simulink model "flyingcap3lvl"  (R2023b)
settings: Solver=ode4  StartTime=0.0  StopTime=0.1  FixedStep=1e-5  RelTol=1e-3  EnableMultiTasking=on
libraries: spsIGBTDiodeLib x12, spsSeriesRLCBranchLib x8, simulink x6, spsVoltageMeasurementLib x4, spsCurrentMeasurementLib x3, spsGroundLib x2, spsDCVoltageSourceLib x1, spsThreePhaseVIMeasurementLib x1, spspowerguiLib x1
settings Model: Creator=Ranit  LastModifiedBy=user
settings SolverCC: AlgebraicLoopSolver=TrustRegion
settings DataIOCC: ReturnWorkspaceOutputs=off
settings OptimizationCC: LifeSpan=inf
settings DebuggingCC: UnconnectedInputMsg=warning  UnconnectedOutputMsg=warning  UnconnectedLineMsg=warning  SFUnexpectedBacktrackingDiag=warning  SFNoUnconditionalDefaultTransitionDiag=warning  ArithmeticOperatorsInVariantConditions=warning
settings ModelReferenceCC: EnableRefExpFcnMdlSchedulingChecks=on
settings SFSimCC: SimUseLocalCustomCode=off  CustomCodeUndefinedFunction=UseInterfaceOnly
settings RTWCC: RTWUseLocalCustomCode=off
settings CodeAppCC: StateflowObjectComments=on
settings GRTTargetCC: TargetLangStandard=C89/C90 (ANSI)
settings ConfigComp: CovMetricSettings=dw  CovSaveCumulativeToWorkspaceVar=on  CovSaveSingleToWorkspaceVar=on  CovExternalEMLEnable=off
settings SimscapeCC: SimscapeNormalizeSystem=off

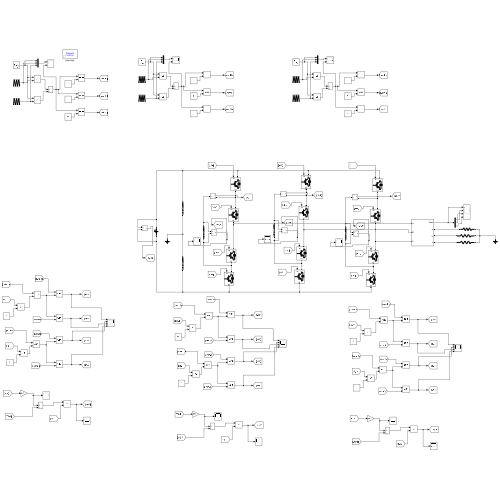
[thumbnail: Simulink's stored preview of the top-level diagram]
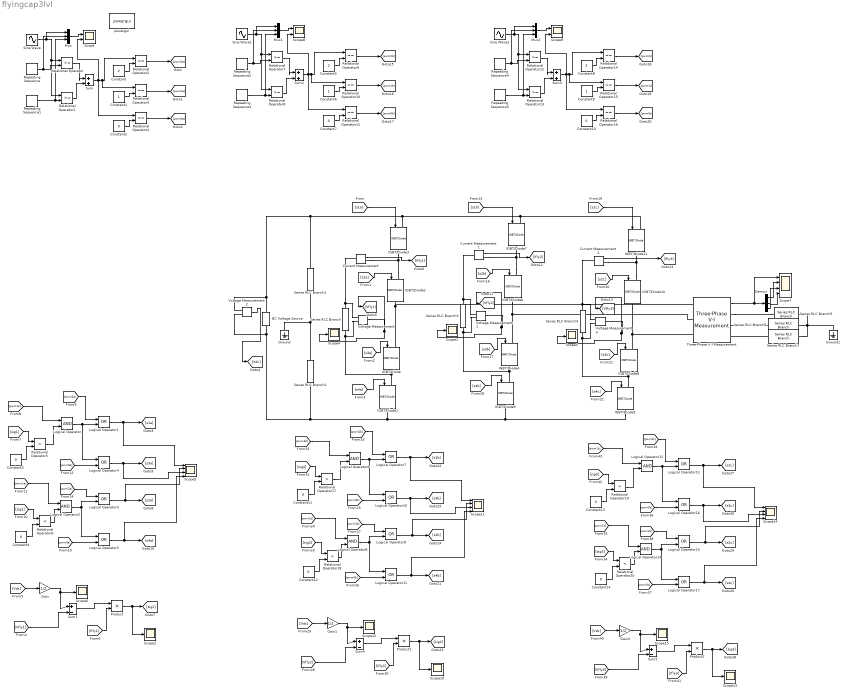
== system flyingcap3lvl ==
  Constant : Constant  Value=2
  Constant1 : Constant
  Constant{2..4,7,10..14} (9 alike) : Constant  Value=0
  Constant5 : Constant  Value=2
  Constant6 : Constant
  Constant8 : Constant  Value=2
  Constant9 : Constant
  Current Measurement : spsCurrentMeasurementLib/Current Measurement  PhasorSimulation=off  OutputType=Complex  PSBequivalent=0
  Current Measurement1 : spsCurrentMeasurementLib/Current Measurement  PhasorSimulation=off  OutputType=Complex  PSBequivalent=0
  Current Measurement2 : spsCurrentMeasurementLib/Current Measurement  PhasorSimulation=off  OutputType=Complex  PSBequivalent=0
  DC Voltage Source : spsDCVoltageSourceLib/DC Voltage Source  Amplitude=100  Measurements=None
  Demux : Demux  Outputs=3
  Gain : Gain  Gain=1/2
  Gain1 : Gain  Gain=1/2
  Gain2 : Gain  Gain=1/2
  Ground : spsGroundLib/Ground  LConnTagsString=a
  Ground1 : spsGroundLib/Ground  LConnTagsString=a
  IGBT/Diode{,1..11} (12 alike) : spsIGBTDiodeLib/IGBT//Diode  Ron=1e-3  Rs=1e5  Cs=inf  Measurements=off
  Logical Operator{,2,6,8,12,14} (6 alike) : Logic  AllPortsSameDT=off  OutDataTypeStr=boolean
  Logical Operator{1,3..5,7,9..11,13,15..17} (12 alike) : Logic  Operator=OR  AllPortsSameDT=off  OutDataTypeStr=boolean
  Mux : Mux  Inputs=3
  Mux1 : Mux  Inputs=3
  Mux2 : Mux  Inputs=3
  Product : Product
  Product1 : Product
  Product2 : Product
  Relational Operator{,1,7..8,12..13} (6 alike) : RelationalOperator  OutDataTypeStr=boolean  InputSameDT=off
  Relational Operator{2..4,9..11,14..16} (9 alike) : RelationalOperator  Operator===  OutDataTypeStr=boolean  InputSameDT=off
  Relational Operator17 : RelationalOperator  Operator=>  OutDataTypeStr=boolean  InputSameDT=off
  Relational Operator18 : RelationalOperator  Operator=<  OutDataTypeStr=boolean  InputSameDT=off
  Relational Operator19 : RelationalOperator  Operator=>  OutDataTypeStr=boolean  InputSameDT=off
  Relational Operator20 : RelationalOperator  Operator=<  OutDataTypeStr=boolean  InputSameDT=off
  Relational Operator5 : RelationalOperator  Operator=>  OutDataTypeStr=boolean  InputSameDT=off
  Relational Operator6 : RelationalOperator  Operator=<  OutDataTypeStr=boolean  InputSameDT=off
  Repeating Sequence : simulink/Sources/Repeating Sequence  rep_seq_t=[0 1 2]*[1/10000]  rep_seq_y=[0 1 0]
  Repeating Sequence1 : simulink/Sources/Repeating Sequence  rep_seq_t=[0 1 2]*[1/10000]  rep_seq_y=[-1 0 -1]
  Repeating Sequence2 : simulink/Sources/Repeating Sequence  rep_seq_t=[0 1 2]*[1/10000]  rep_seq_y=[0 1 0]
  Repeating Sequence3 : simulink/Sources/Repeating Sequence  rep_seq_t=[0 1 2]*[1/10000]  rep_seq_y=[-1 0 -1]
  Repeating Sequence4 : simulink/Sources/Repeating Sequence  rep_seq_t=[0 1 2]*[1/10000]  rep_seq_y=[0 1 0]
  Repeating Sequence5 : simulink/Sources/Repeating Sequence  rep_seq_t=[0 1 2]*[1/10000]  rep_seq_y=[-1 0 -1]
  Scope : Scope  NumInputPorts=2
  Scope{1..4,6,10,12..13,15} (9 alike) : Scope
  Scope{5,7,11,14} (4 alike) : Scope  NumInputPorts=4
  Scope8 : Scope  NumInputPorts=2
  Scope9 : Scope  NumInputPorts=2
  Series RLC Branch{,2..4} (4 alike) : spsSeriesRLCBranchLib/Series RLC Branch  LConnTagsString=__new0  RConnTagsString=__new0  BranchType=RC  Resistance=0.1  Inductance=1e-3  SetiL0=off  InitialCurrent=0  Capacitance=4.7e-3  Setx0=off  InitialVoltage=0  Measurements=None
  Series RLC Branch1 : spsSeriesRLCBranchLib/Series RLC Branch  LConnTagsString=__new0  RConnTagsString=__new0  BranchType=RC  Resistance=0.01  Inductance=1e-3  SetiL0=off  InitialCurrent=0  Capacitance=4.7e-3  Setx0=off  InitialVoltage=0  Measurements=None
  Series RLC Branch5 : spsSeriesRLCBranchLib/Series RLC Branch  LConnTagsString=__new0  RConnTagsString=__new0  BranchType=R  Resistance=500  Inductance=1e-3  SetiL0=off  InitialCurrent=0  Capacitance=1e-6  Setx0=off  InitialVoltage=0  Measurements=Branch voltage
  Series RLC Branch6 : spsSeriesRLCBranchLib/Series RLC Branch  LConnTagsString=__new0  RConnTagsString=__new0  BranchType=R  Resistance=100  Inductance=1e-3  SetiL0=off  InitialCurrent=0  Capacitance=1e-6  Setx0=off  InitialVoltage=0  Measurements=Branch voltage
  Series RLC Branch7 : spsSeriesRLCBranchLib/Series RLC Branch  LConnTagsString=__new0  RConnTagsString=__new0  BranchType=R  Resistance=250  Inductance=1e-3  SetiL0=off  InitialCurrent=0  Capacitance=1e-6  Setx0=off  InitialVoltage=0  Measurements=Branch voltage
  Sine Wave : Sin  Frequency=2*pi*50  SampleTime=0
  Sine Wave1 : Sin  Frequency=2*pi*50  Phase=4*pi/3  SampleTime=0
  Sine Wave2 : Sin  Frequency=2*pi*50  Phase=2*pi/3  SampleTime=0
  Sum : Sum  Inputs=|++
  Sum1 : Sum  Inputs=|+-
  Sum2 : Sum  Inputs=|++
  Sum3 : Sum  Inputs=|++
  Sum4 : Sum  Inputs=|+-
  Sum5 : Sum  Inputs=|+-
  Three-Phase V-I Measurement : spsThreePhaseVIMeasurementLib/Three-Phase V-I Measurement  VoltageMeasurement=phase-to-ground  SetLabelV=off  LabelV=Vabc  Vpu=off  VpuLL=off  CurrentMeasurement=no  SetLabelI=off  LabelI=Iabc  Ipu=off  Pbase=100e6  Vbase=500e3  OutputType=Complex  PhasorSimulation=off  PSBequivalent=0
  Voltage Measurement{,1..3} (4 alike) : spsVoltageMeasurementLib/Voltage Measurement  PhasorSimulation=off  OutputType=Complex  PSBequivalent=0
  powergui : spspowerguiLib/powergui  Priority=1  SimulationMode=Discrete  SampleTime=1e-5  frequency=60  Iterations=50  frequencyindice=0  Pbase=100e6  ErrMax=1e-4  UnitsV=kV  UnitsW=MW  buscounter=0  FunctionMessages=off  echomessages=off  EnableUseOfTLC=off  CurrentSourceSwitches=off  DisableSnubberDevices=off  DisableRonSwitches=off  DisableVfSwitches=off  DisplayEquations=off  AutomaticDiscreteSolvers=off  SolverType=Tustin/Backward Euler (TBE)  Interpol=off  ExternalGateDelay=off  methode=off  Ts=10  x0status=blocks  SPID=off  SwTol=0  HookPort=off  NonlinearTolerance=1e-4  nMaxIteration=100  ContinueOnMaxIteration=off  RestoreLinks=warning  ResistiveCurrentMeasurement=off  Frange=[0:2:500]  Ylog=off  Xlog=on  ShowGrid=off  save=off  variable=ZData  structure=0  ZoomFFT=off  StartTime=0.0  cycles=1  DisplayStyle=1  fundamental=60  FreqAxis=off  MaxFrequency=1000  frequencyindicesteady=1  RmsSteady=1  display=off
  wires:
  Sine Wave/1 -> Mux/1, Relational Operator1/1, Relational Operator/1
  Repeating Sequence/1 -> Mux/2, Relational Operator/2
  Repeating Sequence1/1 -> Mux/3, Relational Operator1/2
  Relational Operator/1 -> Sum/1
  Relational Operator1/1 -> Sum/2
  Mux/1 -> Scope/1
  Constant/1 -> Relational Operator2/2
  Sum/1 -> Scope/2, Relational Operator4/1, Relational Operator3/1, Relational Operator2/1
  Constant1/1 -> Relational Operator3/2
  Constant2/1 -> Relational Operator4/2
  [s1a] -> IGBT/Diode3/1
  [s3a] -> IGBT/Diode/1
  Voltage Measurement2/1 -> [Vdc]
  Voltage Measurement/1 -> Scope4/1, [Vfly1]
  Current Measurement/1 -> [Ifly1]
  [Vdc] -> Gain/1
  Gain/1 -> Scope6/1, Sum1/1
  [Vfly1] -> Sum1/2
  Sum1/1 -> Product/1
  [Ifly1] -> Product/2
  Product/1 -> Scope2/1, [sig1]
  [sig1] -> Relational Operator5/1
  Constant3/1 -> Relational Operator5/2
  Relational Operator2/1 -> [pwm2a]
  Relational Operator3/1 -> [pwm1a]
  Relational Operator4/1 -> [pwm0a]
  Relational Operator5/1 -> Logical Operator/2
  [pwm1a] -> Logical Operator/1
  Logical Operator/1 -> Logical Operator4/1, Logical Operator1/2
  [pwm2a] -> Logical Operator1/1
  [sig1] -> Relational Operator6/1
  Constant4/1 -> Relational Operator6/2
  Relational Operator6/1 -> Logical Operator2/2
  [pwm1a] -> Logical Operator2/1
  Logical Operator1/1 -> Scope5/1, [s1a]
  Logical Operator2/1 -> Logical Operator3/2, Logical Operator5/1
  [pwm0a] -> Logical Operator5/2
  [pwm2a] -> Logical Operator3/1
  [pwm0a] -> Logical Operator4/2
  Logical Operator4/1 -> Scope5/3, [s3a]
  Logical Operator3/1 -> Scope5/2, [s2a]
  Logical Operator5/1 -> Scope5/4, [s4a]
  [s4a] -> IGBT/Diode1/1
  [s2a] -> IGBT/Diode2/1
  [s2b] -> IGBT/Diode6/1
  [s4b] -> IGBT/Diode5/1
  Current Measurement1/1 -> [Ifly2]
  [s1b] -> IGBT/Diode7/1
  [s3b] -> IGBT/Diode4/1
  Voltage Measurement1/1 -> Scope1/1, [Vfly2]
  [s2c] -> IGBT/Diode10/1
  [s4c] -> IGBT/Diode9/1
  Current Measurement2/1 -> [Ifly3]
  [s1c] -> IGBT/Diode11/1
  [s3c] -> IGBT/Diode8/1
  Voltage Measurement3/1 -> Scope3/1, [Vfly3]
  Three-Phase V-I Measurement/1 -> Scope7/1, Demux/1
  Constant7/1 -> Relational Operator11/2
  Repeating Sequence3/1 -> Mux1/3, Relational Operator8/2
  Relational Operator11/1 -> [pwm0b]
  Relational Operator10/1 -> [pwm1b]
  Relational Operator7/1 -> Sum2/1
  Relational Operator9/1 -> [pwm2b]
  Constant6/1 -> Relational Operator10/2
  Relational Operator8/1 -> Sum2/2
  Mux1/1 -> Scope8/1
  Repeating Sequence2/1 -> Mux1/2, Relational Operator7/2
  Constant5/1 -> Relational Operator9/2
  Sum2/1 -> Scope8/2, Relational Operator11/1, Relational Operator10/1, Relational Operator9/1
  Sine Wave1/1 -> Mux1/1, Relational Operator8/1, Relational Operator7/1
  Constant10/1 -> Relational Operator16/2
  Repeating Sequence5/1 -> Mux2/3, Relational Operator13/2
  Relational Operator16/1 -> [pwm0c]
  Relational Operator15/1 -> [pwm1c]
  Relational Operator12/1 -> Sum3/1
  Relational Operator14/1 -> [pwm2c]
  Constant9/1 -> Relational Operator15/2
  Relational Operator13/1 -> Sum3/2
  Mux2/1 -> Scope9/1
  Repeating Sequence4/1 -> Mux2/2, Relational Operator12/2
  Constant8/1 -> Relational Operator14/2
  Sum3/1 -> Scope9/2, Relational Operator16/1, Relational Operator15/1, Relational Operator14/1
  Sine Wave2/1 -> Mux2/1, Relational Operator13/1, Relational Operator12/1
  [pwm0b] -> Logical Operator11/2
  Logical Operator11/1 -> Scope11/4, [s4b]
  [pwm1b] -> Logical Operator8/1
  [Ifly2] -> Product1/2
  Relational Operator17/1 -> Logical Operator6/2
  Logical Operator7/1 -> Scope11/1, [s1b]
  Logical Operator10/1 -> Scope11/3, [s3b]
  [Vfly2] -> Sum4/2
  Logical Operator8/1 -> Logical Operator9/2, Logical Operator11/1
  [sig2] -> Relational Operator18/1
  Relational Operator18/1 -> Logical Operator8/2
  [pwm0b] -> Logical Operator10/2
  [pwm2b] -> Logical Operator9/1
  [pwm2b] -> Logical Operator7/1
  Logical Operator6/1 -> Logical Operator10/1, Logical Operator7/2
  Constant12/1 -> Relational Operator18/2
  Logical Operator9/1 -> Scope11/2, [s2b]
  Constant11/1 -> Relational Operator17/2
  [Vdc] -> Gain1/1
  [sig2] -> Relational Operator17/1
  Gain1/1 -> Scope12/1, Sum4/1
  Sum4/1 -> Product1/1
  Product1/1 -> Scope10/1, [sig2]
  [pwm1b] -> Logical Operator6/1
  [pwm0c] -> Logical Operator17/2
  Logical Operator17/1 -> Scope14/4, [s4c]
  [pwm1c] -> Logical Operator14/1
  [Ifly3] -> Product2/2
  Relational Operator19/1 -> Logical Operator12/2
  Logical Operator13/1 -> Scope14/1, [s1c]
  Logical Operator16/1 -> Scope14/3, [s3c]
  [Vfly3] -> Sum5/2
  Logical Operator14/1 -> Logical Operator15/2, Logical Operator17/1
  [sig3] -> Relational Operator20/1
  Relational Operator20/1 -> Logical Operator14/2
  [pwm0c] -> Logical Operator16/2
  [pwm2c] -> Logical Operator15/1
  [pwm2c] -> Logical Operator13/1
  Logical Operator12/1 -> Logical Operator16/1, Logical Operator13/2
  Constant14/1 -> Relational Operator20/2
  Logical Operator15/1 -> Scope14/2, [s2c]
  Constant13/1 -> Relational Operator19/2
  [Vdc] -> Gain2/1
  [sig3] -> Relational Operator19/1
  Gain2/1 -> Scope15/1, Sum5/1
  Sum5/1 -> Product2/1
  Product2/1 -> Scope13/1, [sig3]
  [pwm1c] -> Logical Operator12/1
  Demux/1 -> Scope7/2
  Demux/2 -> Scope7/3
  Demux/3 -> Scope7/4
  connections:
  Current Measurement/RConn1 -- IGBT/Diode3/RConn1 -- IGBT/Diode2/LConn1
  IGBT/Diode2/RConn1 -- Three-Phase V-I Measurement/LConn1 -- IGBT/Diode/LConn1
  Voltage Measurement/LConn2 -- IGBT/Diode1/LConn1 -- IGBT/Diode/RConn1 -- Series RLC Branch/RConn1
  Series RLC Branch/LConn1 -- Voltage Measurement/LConn1 -- Current Measurement/LConn1
  Series RLC Branch2/LConn1 -- Ground/LConn1 -- Series RLC Branch1/RConn1
  Series RLC Branch1/LConn1 -- IGBT/Diode11/LConn1 -- IGBT/Diode7/LConn1 -- IGBT/Diode3/LConn1 -- Voltage Measurement2/LConn1 -- DC Voltage Source/RConn1
  Series RLC Branch2/RConn1 -- Voltage Measurement2/LConn2 -- DC Voltage Source/LConn1 -- IGBT/Diode1/RConn1 -- IGBT/Diode5/RConn1 -- IGBT/Diode9/RConn1
  IGBT/Diode6/LConn1 -- Current Measurement1/RConn1 -- IGBT/Diode7/RConn1
  Current Measurement1/LConn1 -- Series RLC Branch3/LConn1 -- Voltage Measurement1/LConn1
  IGBT/Diode4/RConn1 -- Voltage Measurement1/LConn2 -- Series RLC Branch3/RConn1 -- IGBT/Diode5/LConn1
  IGBT/Diode6/RConn1 -- Three-Phase V-I Measurement/LConn2 -- IGBT/Diode4/LConn1
  IGBT/Diode10/LConn1 -- Current Measurement2/RConn1 -- IGBT/Diode11/RConn1
  Current Measurement2/LConn1 -- Series RLC Branch4/LConn1 -- Voltage Measurement3/LConn1
  IGBT/Diode8/RConn1 -- Voltage Measurement3/LConn2 -- Series RLC Branch4/RConn1 -- IGBT/Diode9/LConn1
  IGBT/Diode10/RConn1 -- Three-Phase V-I Measurement/LConn3 -- IGBT/Diode8/LConn1
  Series RLC Branch6/RConn1 -- Series RLC Branch5/RConn1 -- Ground1/LConn1 -- Series RLC Branch7/RConn1
  Three-Phase V-I Measurement/RConn1 -- Series RLC Branch5/LConn1
  Series RLC Branch7/LConn1 -- Three-Phase V-I Measurement/RConn3
  Three-Phase V-I Measurement/RConn2 -- Series RLC Branch6/LConn1
